simulink model "boatlab_5_d"  (R2017a)
settings: Solver=ode45  StartTime=0.0  StopTime=sim_time  RelTol=1e-3  EnableMultiTasking=on
values from neighbouring files (symbols this model uses):
  ref = 30    [boatlab_5_5_full.m]    (also in boatlab_5_5a.m)
  Ts = 1/Fs    (= 0.1)    [boatlab_5_5_full.m]    (also in boatlab_5_5a.m)
libraries: simulink x2, cstblocks x1
settings Model: Creator=markh  LastModifiedBy=evenwa
settings DataIOCC: LimitDataPoints=on  SaveFormat=Array  SignalLoggingSaveFormat=ModelDataLogs  SignalLoggingName=sigsOut
settings OptimizationCC: InitFltsAndDblsToZero=on  LifeSpan=inf
settings DebuggingCC: SaveWithParameterizedLinksMsg=none  UnderspecifiedInitializationDetection=Classic  MergeDetectMultiDrivingBlocksExec=none  SignalResolutionControl=TryResolveAllWithWarning  MultiTaskDSMMsg=warning  MultiTaskCondExecSysMsg=none  FcnCallInpInsideContextMsg=warning  StateNameClashWarn=warning  SFUnexpectedBacktrackingDiag=warning  SFNoUnconditionalDefaultTransitionDiag=warning  SFExecutionAtInitializationDiag=none
settings HardwareCC: ProdBitPerPointer=32  ProdBitPerSizeT=32  ProdBitPerPtrDiffT=32  ProdLargestAtomicFloat=None  ProdIntDivRoundTo=Undefined  ProdEndianess=Unspecified  ProdWordSize=32  ProdHWDeviceType=32-bit Generic  TargetUnknown=on
settings ModelReferenceCC: PropagateSignalLabelsOutOfModel=off
settings GRTTargetCC: TargetFcnLib=ansi_tfl_tmw.mat  TargetLangStandard=C89/C90 (ANSI)  GeneratePreprocessorConditionals=Disable all  CombineOutputUpdateFcns=off  GRTInterface=on
settings ConfigComp: CovMetricSettings=dw  CovHtmlReporting=on  CovSaveCumulativeToWorkspaceVar=on  CovSaveSingleToWorkspaceVar=on  CovExternalEMLEnable=off

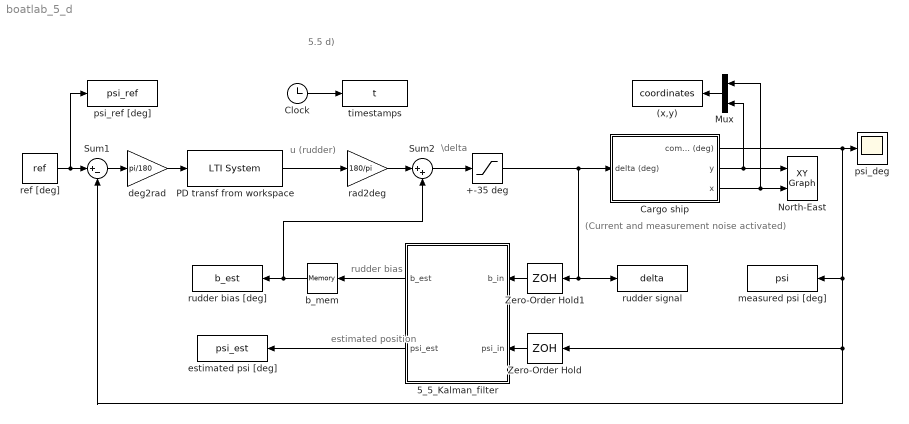
== system boatlab_5_d ==
  note: u (rudder)
  note: 5.5 d)
  note: (Current and measurement noise activated)
  note: rudder bias
  note: estimated position
  note: \delta
  " +-35 deg" : Saturate  UpperLimit=35  LowerLimit=-35
  (x,y) : ToWorkspace  VariableName=coordinates  SampleTime=-1
  5_5_Kalman_filter : MATLAB Function  TreatAsAtomicUnit=on
  Cargo ship : Subsystem  mask(Simple shipmodel for a cargo ship){noise=on, current=on, logic=off}
      mask prompts: noise "measurement noise"; logic "waves"
      mask help:
      | Measurement noise:
      | 	checked = noise on
      | 	unchecked = noise off
      |
      | Current:
      | 	checked = current on
      | 	unchecked = current off
      |
      | Waves:
      | 	checked = waves on
      | 	unchecked = waves off
      |
      | Author: Jørgen Spjøtvold, 9/10-2003
      | TTK 4115 Linear system theory.
      | Modified by Jostein Bakkeheim 26/10-2006
  Clock : Clock
  Mux : Mux  Inputs=2
  North-East : simulink/Sinks/XY Graph  xmin=-5000  xmax=5000  ymin=-5000  ymax=5000  st=-1
  PD transf from workspace : cstblocks/LTI System  sys=tf(num, den)  IC=[]
  Sum1 : Sum  Inputs=|+-
  Sum2 : Sum  Inputs=|++
  Zero-Order Hold : ZeroOrderHold  SampleTime=Ts
  Zero-Order Hold1 : ZeroOrderHold  SampleTime=Ts
  b_mem : Memory
  deg2rad : Gain  Gain=pi/180
  estimated psi [deg] : ToWorkspace  VariableName=psi_est  SampleTime=-1
  measured psi [deg] : ToWorkspace  VariableName=psi  SampleTime=-1
  psi_deg : Scope
  psi_ref [deg] : ToWorkspace  VariableName=psi_ref  SampleTime=-1
  rad2deg : Gain  Gain=180/pi
  ref [deg] : Constant  Value=ref
  rudder bias [deg] : ToWorkspace  VariableName=b_est  SampleTime=-1
  rudder signal : ToWorkspace  VariableName=delta  SampleTime=-1
  timestamps : ToWorkspace  VariableName=t  SampleTime=-1
  wires:
  Cargo ship/3(x) -> Mux/1, North-East/2
  Cargo ship/2(y) -> Mux/2, North-East/1
  Clock/1 -> timestamps/1
  5_5_Kalman_filter/1(b_est) -> b_mem/1
  Zero-Order Hold/1 -> 5_5_Kalman_filter/2(psi_in)
  Zero-Order Hold1/1 -> 5_5_Kalman_filter/1(b_in)
  Mux/1 -> (x,y)/1
  b_mem/1 -> rudder bias [deg]/1, Sum2/2
  5_5_Kalman_filter/2(psi_est) -> estimated psi [deg]/1
  ref [deg]/1 -> psi_ref [deg]/1, Sum1/1
  Sum1/1 -> deg2rad/1
  deg2rad/1 -> PD transf from workspace/1
  " +-35 deg"/1 -> rudder signal/1, Zero-Order Hold1/1, Cargo ship/1(delta (deg))
  Sum2/1 -> " +-35 deg"/1
  rad2deg/1 -> Sum2/1
  PD transf from workspace/1 -> rad2deg/1
  Cargo ship/1(compass (deg)) -> Sum1/2, Zero-Order Hold/1, measured psi [deg]/1, psi_deg/1

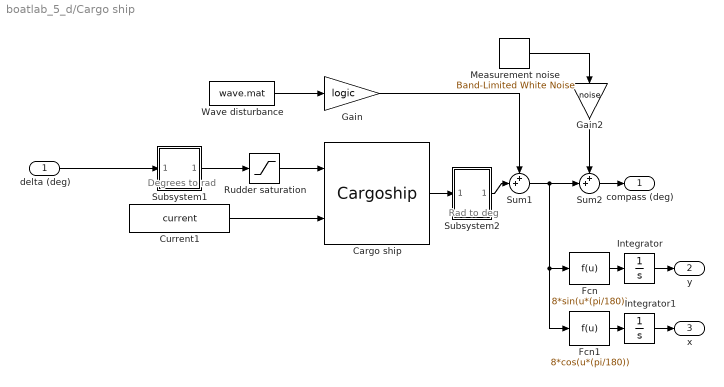
== system boatlab_5_d/Cargo ship ==
  note: Degrees to rad
  note: Rad to deg
  delta (deg) : Inport
  Cargo ship : S-Function  FunctionName=Cargoship  SFunctionDeploymentMode=off  EnableBusSupport=off  mask(Cargo ship){}
      mask help:
      | S-function which simulates a cargo ship.
      |
      | Author: Jørgen Spjøtvold
      | 20.10-2003
      | Modified by Jostein Bakkeheim 27.10.2006
  Current1 : Constant  Value=current
  Fcn : Fcn  Expr=8*sin(u*(pi/180))
  Fcn1 : Fcn  Expr=8*cos(u*(pi/180))
  Gain : Gain  Gain=logic  SaturateOnIntegerOverflow=on  OutDataTypeStr=Inherit: Same as input  ParamDataTypeStr=Inherit: Same as input
  Gain2 : Gain  Gain=noise  SaturateOnIntegerOverflow=on  OutDataTypeStr=Inherit: Same as input  ParamDataTypeStr=Inherit: Same as input
  Integrator : Integrator
  Integrator1 : Integrator
  Measurement noise : simulink/Sources/Band-Limited White Noise  Cov=[0.001]  Ts=.5  seed=[23341]
  Rudder saturation : Saturate  UpperLimit=45*(pi/180)  LowerLimit=-45*(pi/180)
  Subsystem1 : Subsystem  mask(degrees to radians){}
      mask help: Converts degrees to radians
      mask Display: fprintf('D2R');
  Subsystem2 : Subsystem  mask(radians to degrees){}
      mask help: Converts radians to degrees
      mask Display: fprintf('R2D');
  Sum1 : Sum  Inputs=++|  SaturateOnIntegerOverflow=on
  Sum2 : Sum  Inputs=++|  SaturateOnIntegerOverflow=on
  Wave disturbance : FromFile  FileName=wave.mat  SampleTime=0
  compass (deg) : Outport
  y : Outport  Port=2
  x : Outport  Port=3
  wires:
  delta (deg)/1 -> Subsystem1/1(In1)
  Fcn/1 -> Integrator/1
  Integrator/1 -> y/1
  Fcn1/1 -> Integrator1/1
  Integrator1/1 -> x/1
  Wave disturbance/1 -> Gain/1
  Subsystem2/1(Out1) -> Sum1/2
  Gain/1 -> Sum1/1
  Sum1/1 -> Fcn/1, Fcn1/1, Sum2/2
  Cargo ship/1 -> Subsystem2/1(In1)
  Subsystem1/1(Out1) -> Rudder saturation/1
  Rudder saturation/1 -> Cargo ship/1
  Sum2/1 -> compass (deg)/1
  Measurement noise/1 -> Gain2/1
  Gain2/1 -> Sum2/1
  Current1/1 -> Cargo ship/2

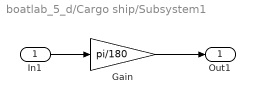
== system boatlab_5_d/Cargo ship/Subsystem1 ==
  In1 : Inport
  Gain : Gain  Gain=pi/180  SaturateOnIntegerOverflow=on  OutDataTypeStr=Inherit: Same as input  ParamDataTypeStr=Inherit: Same as input
  Out1 : Outport
  wires:
  Gain/1 -> Out1/1
  In1/1 -> Gain/1

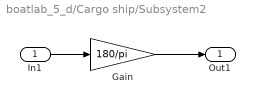
== system boatlab_5_d/Cargo ship/Subsystem2 ==
  In1 : Inport
  Gain : Gain  Gain=180/pi  SaturateOnIntegerOverflow=on  OutDataTypeStr=Inherit: Same as input  ParamDataTypeStr=Inherit: Same as input
  Out1 : Outport
  wires:
  Gain/1 -> Out1/1
  In1/1 -> Gain/1

== matlab function boatlab_5_d/5_5_Kalman_filter ==
  data: b_est output; b_in input; psi_est output; psi_in input; data parameter
% @b_k:       rudder angle control signal 
% @psi_k:     measured compass angle 
% @data:      structure containing initialization values
% returns:
% @b_est:     estimated rudder angle bias
% @psi_est:   estimated compass angle
% the init_data will be kept persistent while in loop
function [b_est, psi_est] = kalman_filter(b_in, psi_in, data)
%#codegen

persistent init_flag x_pri P_pri Ad Bd Ed Cd Q R I;
if isempty(init_flag)
    init_flag = 1;
    % distribute copies of init_data
    [x_pri,P_pri,Ad,Bd,Ed,Cd,Q,R,I] = deal(data.x_pri0, data.P_pri0, ... 
        data.Ad, data.Bd, data.Ed, data.Cd, data.Q, data.R, data.I);
end

% 1. compute Kalman gain:
L = (P_pri*Cd')/((Cd*P_pri*Cd'+R));      % 5x1

% 2. Update estimate with measurement (posteriori):
x_post = x_pri + L*(psi_in-Cd*x_pri);    % 5x1

% 3. Compute error variance for updated estimate:
P = (I - L*Cd)*P_pri*(I-L*Cd)' + L*R*L'; % 5x5

% 4. Project ahead (priori)
x_pri = Ad*x_post + Bd*b_in;             % 5x1
P_pri = Ad*P*Ad' + Ed*Q*Ed';               % 5x5

% output: row 3 and 5 of estimated states
psi_est = x_post(3); b_est = x_post(5);
